simulink model "gm_dac_spi"  (R2022a)
settings: Solver=FixedStepDiscrete  StartTime=0.0  StopTime=1000/100e6  RelTol=1e-3
libraries: hdlsllib x152, simulink x1
settings Model: Creator=ts  LastModifiedBy=ts
settings SolverCC: AlgebraicLoopSolver=TrustRegion
settings DataIOCC: LimitDataPoints=on  SaveOutput=off  SaveTime=off
settings OptimizationCC: BlockReduction=off  ConditionallyExecuteInputs=off  DefaultParameterBehavior=Inlined  LifeSpan=inf
settings DebuggingCC: AlgebraicLoopMsg=error  InheritedTsInSrcMsg=none  SingleTaskRateTransMsg=error  UnconnectedInputMsg=warning  UnconnectedOutputMsg=warning  UnconnectedLineMsg=warning  AllowSymbolicDim=off  StrictBusMsg=ErrorOnBusTreatedAsVector  SFUnexpectedBacktrackingDiag=warning  SFNoUnconditionalDefaultTransitionDiag=warning  SFExecutionAtInitializationDiag=none  SFMachineParentedDataDiag=warning  ArithmeticOperatorsInVariantConditions=warning
settings HardwareCC: ProdBitPerPointer=32  ProdBitPerSizeT=32  ProdBitPerPtrDiffT=32  ProdLargestAtomicFloat=None  ProdIntDivRoundTo=Undefined  ProdEndianess=Unspecified  ProdWordSize=32  ProdHWDeviceType=ASIC/FPGA->ASIC/FPGA  ProdEqTarget=off
settings SFSimCC: SimUseLocalCustomCode=off  CustomCodeUndefinedFunction=UseInterfaceOnly
settings RTWCC: RTWUseLocalCustomCode=off
settings CodeAppCC: StateflowObjectComments=on
settings GRTTargetCC: TargetLangStandard=C89/C90 (ANSI)
settings ConfigComp: CovScope=ReferencedModels  CovMetricSettings=dw  CovSaveCumulativeToWorkspaceVar=on  CovSaveSingleToWorkspaceVar=on  CovExternalEMLEnable=off  CovSFcnEnable=off

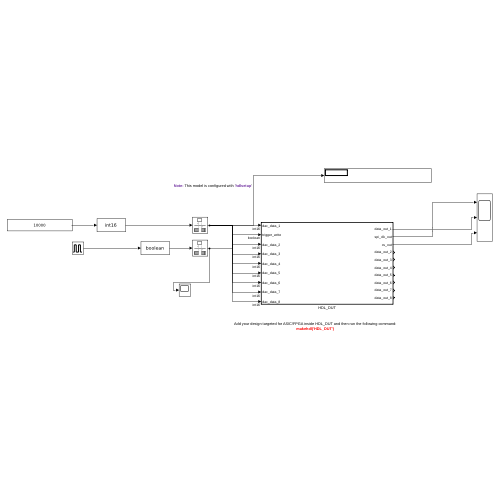
[thumbnail: Simulink's stored preview of the top-level diagram]
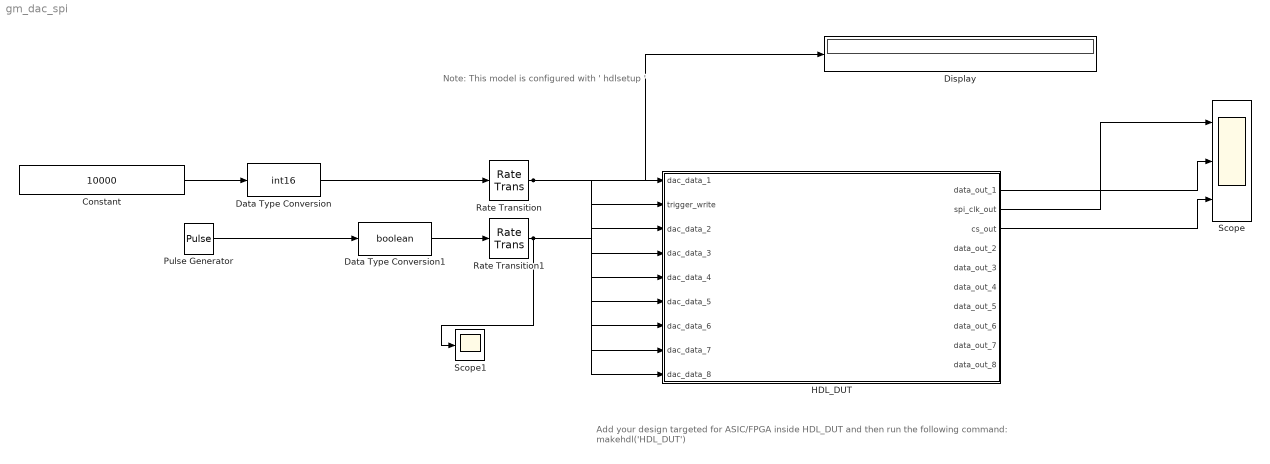
== system gm_dac_spi ==
  note: Add your design targeted for ASIC/FPGA inside HDL_DUT and then run the following command:
      | makehdl('HDL_DUT')
  note: Note: This model is configured with ' hdlsetup '
  Constant : Constant  Value=10000  OutDataTypeStr=int16  SampleTime=1/100e6
  Data Type Conversion : DataTypeConversion  OutDataTypeStr=int16  SaturateOnIntegerOverflow=off  RndMeth=Floor
  Data Type Conversion1 : DataTypeConversion  OutDataTypeStr=boolean  SaturateOnIntegerOverflow=off  RndMeth=Floor
  Display : Display
      settings: Format=binary (Stored Integer)
  HDL_DUT : Subsystem  TreatAsAtomicUnit=on
  Pulse Generator : DiscretePulseGenerator  PulseType=Time based  Period=200/100e6  PulseWidth=10
  Rate Transition : RateTransition  OutPortSampleTime=1/100e6
  Rate Transition1 : RateTransition  OutPortSampleTime=1/100e6
  Scope : Scope  NumInputPorts=3
  Scope1 : Scope
  wires:
  Pulse Generator/1 -> Data Type Conversion1/1
  Data Type Conversion1/1 -> Rate Transition1/1
  Rate Transition1/1 -> HDL_DUT/2(trigger_write), Scope1/1
  HDL_DUT/2(spi_clk_out) -> Scope/1
  HDL_DUT/3(cs_out) -> Scope/3
  Rate Transition/1 -> HDL_DUT/1(dac_data_1), HDL_DUT/3(dac_data_2), HDL_DUT/4(dac_data_3), HDL_DUT/5(dac_data_4), HDL_DUT/6(dac_data_5), HDL_DUT/7(dac_data_6), HDL_DUT/8(dac_data_7), HDL_DUT/9(dac_data_8), Display/1
  Data Type Conversion/1 -> Rate Transition/1
  HDL_DUT/1(data_out_1) -> Scope/2
  Constant/1 -> Data Type Conversion/1

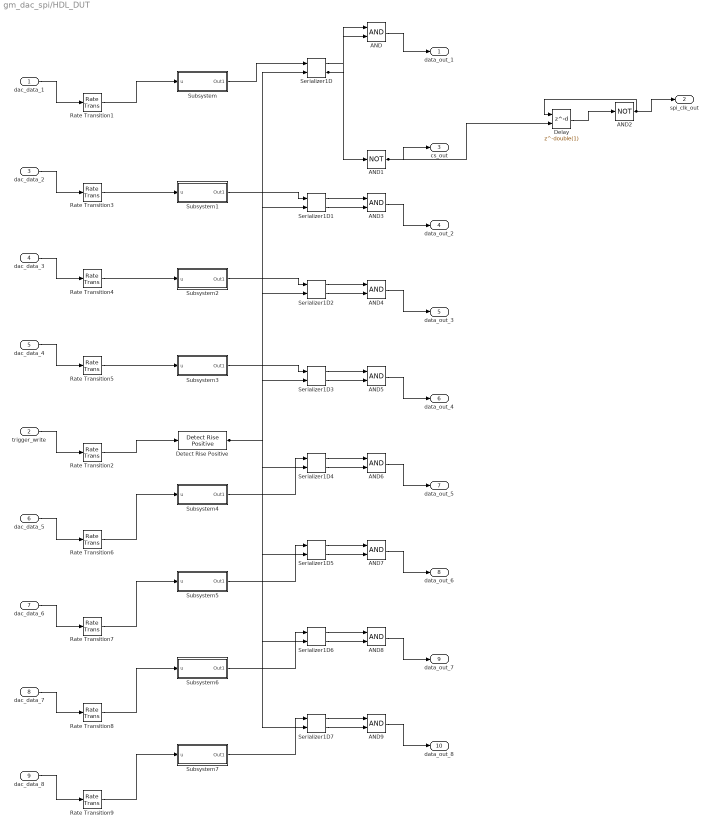
== system gm_dac_spi/HDL_DUT ==
  dac_data_1 : Inport  OutDataTypeStr=int16  PortDimensions=1  SampleTime=1e-08
  trigger_write : Inport  Port=2  OutDataTypeStr=boolean  PortDimensions=1  SampleTime=1e-08
  dac_data_2 : Inport  Port=3  OutDataTypeStr=int16  PortDimensions=1  SampleTime=1e-08
  dac_data_3 : Inport  Port=4  OutDataTypeStr=int16  PortDimensions=1  SampleTime=1e-08
  dac_data_4 : Inport  Port=5  OutDataTypeStr=int16  PortDimensions=1  SampleTime=1e-08
  dac_data_5 : Inport  Port=6  OutDataTypeStr=int16  PortDimensions=1  SampleTime=1e-08
  dac_data_6 : Inport  Port=7  OutDataTypeStr=int16  PortDimensions=1  SampleTime=1e-08
  dac_data_7 : Inport  Port=8  OutDataTypeStr=int16  PortDimensions=1  SampleTime=1e-08
  dac_data_8 : Inport  Port=9  OutDataTypeStr=int16  PortDimensions=1  SampleTime=1e-08
  AND{,3..9} (8 alike) : Logic  AllPortsSameDT=off  OutDataTypeStr=boolean  SampleTime=1e-08
  AND1 : Logic  Operator=NOT  Inputs=1  AllPortsSameDT=off  OutDataTypeStr=boolean  SampleTime=1e-08
  AND2 : Logic  Operator=NOT  Inputs=1  AllPortsSameDT=off  OutDataTypeStr=boolean  SampleTime=1e-08
  Delay : Delay  DelayLength=double(1)  InitialCondition=1  ExternalReset=Level
      settings: InputPortMap=u0,r5
  Detect Rise Positive : simulink/Logic and Bit Operations/Detect Rise Positive  vinit=0  OutDataTypeStr=boolean
  Rate Transition{1..9} (9 alike) : RateTransition  InitialCondition=double(0)  OutPortSampleTimeOpt=Multiple of input port sample time  OutPortSampleTimeMultiple=32
  Serializer1D{,1..7} (8 alike) : hdlsllib/HDL Operations/Serializer1D  Ratio=32  IdleCycles=0  validIn=on  startOut=off  validOut=on  inputDataDimensions=32  inputSampleTime=3.2e-07  inputSignalType=real
      settings: SourceProductBaseCode=SL
  Subsystem : Subsystem
  Subsystem1 : Subsystem
  Subsystem2 : Subsystem
  Subsystem3 : Subsystem
  Subsystem4 : Subsystem
  Subsystem5 : Subsystem
  Subsystem6 : Subsystem
  Subsystem7 : Subsystem
  data_out_1 : Outport  SampleTime=1e-08  VectorParamsAs1DForOutWhenUnconnected=off
  spi_clk_out : Outport  Port=2  SampleTime=1e-08
  cs_out : Outport  Port=3  SampleTime=1e-08
  data_out_2 : Outport  Port=4  SampleTime=1e-08  VectorParamsAs1DForOutWhenUnconnected=off
  data_out_3 : Outport  Port=5  SampleTime=1e-08  VectorParamsAs1DForOutWhenUnconnected=off
  data_out_4 : Outport  Port=6  SampleTime=1e-08  VectorParamsAs1DForOutWhenUnconnected=off
  data_out_5 : Outport  Port=7  SampleTime=1e-08  VectorParamsAs1DForOutWhenUnconnected=off
  data_out_6 : Outport  Port=8  SampleTime=1e-08  VectorParamsAs1DForOutWhenUnconnected=off
  data_out_7 : Outport  Port=9  SampleTime=1e-08  VectorParamsAs1DForOutWhenUnconnected=off
  data_out_8 : Outport  Port=10  SampleTime=1e-08  VectorParamsAs1DForOutWhenUnconnected=off
  wires:
  dac_data_1/1 -> Rate Transition1/1
  trigger_write/1 -> Rate Transition2/1
  dac_data_2/1 -> Rate Transition3/1
  dac_data_3/1 -> Rate Transition4/1
  dac_data_4/1 -> Rate Transition5/1
  dac_data_5/1 -> Rate Transition6/1
  dac_data_6/1 -> Rate Transition7/1
  dac_data_7/1 -> Rate Transition8/1
  dac_data_8/1 -> Rate Transition9/1
  AND/1 -> data_out_1/1
  AND1/1 -> Delay/2, cs_out/1
  AND2/1 -> Delay/1, spi_clk_out/1
  AND3/1 -> data_out_2/1
  AND4/1 -> data_out_3/1
  AND5/1 -> data_out_4/1
  AND6/1 -> data_out_5/1
  AND7/1 -> data_out_6/1
  AND8/1 -> data_out_7/1
  AND9/1 -> data_out_8/1
  Delay/1 -> AND2/1
  Detect Rise Positive/1 -> Serializer1D7/2, Serializer1D6/2, Serializer1D5/2, Serializer1D4/2, Serializer1D3/2, Serializer1D2/2, Serializer1D1/2, Serializer1D/2
  Rate Transition1/1 -> Subsystem/1(u)
  Rate Transition2/1 -> Detect Rise Positive/1
  Rate Transition3/1 -> Subsystem1/1(u)
  Rate Transition4/1 -> Subsystem2/1(u)
  Rate Transition5/1 -> Subsystem3/1(u)
  Rate Transition6/1 -> Subsystem4/1(u)
  Rate Transition7/1 -> Subsystem5/1(u)
  Rate Transition8/1 -> Subsystem6/1(u)
  Rate Transition9/1 -> Subsystem7/1(u)
  Serializer1D/1 -> AND/1
  Serializer1D/2 -> AND1/1, AND/2
  Serializer1D1/1 -> AND3/1
  Serializer1D1/2 -> AND3/2
  Serializer1D2/1 -> AND4/1
  Serializer1D2/2 -> AND4/2
  Serializer1D3/1 -> AND5/1
  Serializer1D3/2 -> AND5/2
  Serializer1D4/1 -> AND6/1
  Serializer1D4/2 -> AND6/2
  Serializer1D5/1 -> AND7/1
  Serializer1D5/2 -> AND7/2
  Serializer1D6/1 -> AND8/1
  Serializer1D6/2 -> AND8/2
  Serializer1D7/1 -> AND9/1
  Serializer1D7/2 -> AND9/2
  Subsystem/1(Out1) -> Serializer1D/1
  Subsystem1/1(Out1) -> Serializer1D1/1
  Subsystem2/1(Out1) -> Serializer1D2/1
  Subsystem3/1(Out1) -> Serializer1D3/1
  Subsystem4/1(Out1) -> Serializer1D4/1
  Subsystem5/1(Out1) -> Serializer1D5/1
  Subsystem6/1(Out1) -> Serializer1D6/1
  Subsystem7/1(Out1) -> Serializer1D7/1

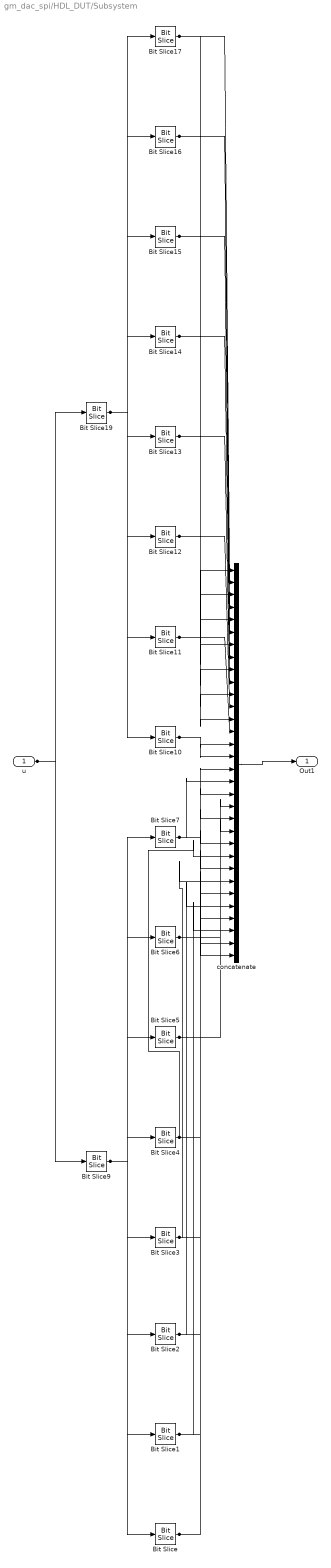
== system gm_dac_spi/HDL_DUT/Subsystem ==
  u : Inport  OutDataTypeStr=int16  PortDimensions=1  SampleTime=3.2e-07
  Bit Slice : hdlsllib/Logic and Bit Operations/Bit Slice  lidx=double(0)  ridx=double(0)
      settings: SourceProductBaseCode=SL
  Bit Slice1 : hdlsllib/Logic and Bit Operations/Bit Slice  lidx=double(1)  ridx=double(1)
      settings: SourceProductBaseCode=SL
  Bit Slice10 : hdlsllib/Logic and Bit Operations/Bit Slice  lidx=double(0)  ridx=double(0)
      settings: SourceProductBaseCode=SL
  Bit Slice11 : hdlsllib/Logic and Bit Operations/Bit Slice  lidx=double(1)  ridx=double(1)
      settings: SourceProductBaseCode=SL
  Bit Slice12 : hdlsllib/Logic and Bit Operations/Bit Slice  lidx=double(2)  ridx=double(2)
      settings: SourceProductBaseCode=SL
  Bit Slice13 : hdlsllib/Logic and Bit Operations/Bit Slice  lidx=double(3)  ridx=double(3)
      settings: SourceProductBaseCode=SL
  Bit Slice14 : hdlsllib/Logic and Bit Operations/Bit Slice  lidx=double(4)  ridx=double(4)
      settings: SourceProductBaseCode=SL
  Bit Slice15 : hdlsllib/Logic and Bit Operations/Bit Slice  lidx=double(5)  ridx=double(5)
      settings: SourceProductBaseCode=SL
  Bit Slice16 : hdlsllib/Logic and Bit Operations/Bit Slice  lidx=double(6)  ridx=double(6)
      settings: SourceProductBaseCode=SL
  Bit Slice17 : hdlsllib/Logic and Bit Operations/Bit Slice  lidx=double(7)  ridx=double(7)
      settings: SourceProductBaseCode=SL
  Bit Slice19 : hdlsllib/Logic and Bit Operations/Bit Slice  lidx=double(15)  ridx=double(8)
      settings: SourceProductBaseCode=SL
  Bit Slice2 : hdlsllib/Logic and Bit Operations/Bit Slice  lidx=double(2)  ridx=double(2)
      settings: SourceProductBaseCode=SL
  Bit Slice3 : hdlsllib/Logic and Bit Operations/Bit Slice  lidx=double(3)  ridx=double(3)
      settings: SourceProductBaseCode=SL
  Bit Slice4 : hdlsllib/Logic and Bit Operations/Bit Slice  lidx=double(4)  ridx=double(4)
      settings: SourceProductBaseCode=SL
  Bit Slice5 : hdlsllib/Logic and Bit Operations/Bit Slice  lidx=double(5)  ridx=double(5)
      settings: SourceProductBaseCode=SL
  Bit Slice6 : hdlsllib/Logic and Bit Operations/Bit Slice  lidx=double(6)  ridx=double(6)
      settings: SourceProductBaseCode=SL
  Bit Slice7 : hdlsllib/Logic and Bit Operations/Bit Slice  lidx=double(7)  ridx=double(7)
      settings: SourceProductBaseCode=SL
  Bit Slice9 : hdlsllib/Logic and Bit Operations/Bit Slice  lidx=double(7)  ridx=double(0)
      settings: SourceProductBaseCode=SL
  concatenate : Concatenate  NumInputs=32
  Out1 : Outport  SampleTime=3.2e-07
  wires:
  u/1 -> Bit Slice9/1, Bit Slice19/1
  Bit Slice/1 -> concatenate/32, concatenate/31
  Bit Slice1/1 -> concatenate/30, concatenate/29
  Bit Slice10/1 -> concatenate/16, concatenate/15
  Bit Slice11/1 -> concatenate/14, concatenate/13
  Bit Slice12/1 -> concatenate/12, concatenate/11
  Bit Slice13/1 -> concatenate/10, concatenate/9
  Bit Slice14/1 -> concatenate/8, concatenate/7
  Bit Slice15/1 -> concatenate/6, concatenate/5
  Bit Slice16/1 -> concatenate/4, concatenate/3
  Bit Slice17/1 -> concatenate/2, concatenate/1
  Bit Slice19/1 -> Bit Slice17/1, Bit Slice16/1, Bit Slice15/1, Bit Slice14/1, Bit Slice13/1, Bit Slice12/1, Bit Slice11/1, Bit Slice10/1
  Bit Slice2/1 -> concatenate/28, concatenate/27
  Bit Slice3/1 -> concatenate/26, concatenate/25
  Bit Slice4/1 -> concatenate/24, concatenate/23
  Bit Slice5/1 -> concatenate/22, concatenate/21
  Bit Slice6/1 -> concatenate/20, concatenate/19
  Bit Slice7/1 -> concatenate/18, concatenate/17
  Bit Slice9/1 -> Bit Slice7/1, Bit Slice6/1, Bit Slice5/1, Bit Slice4/1, Bit Slice3/1, Bit Slice2/1, Bit Slice1/1, Bit Slice/1
  concatenate/1 -> Out1/1

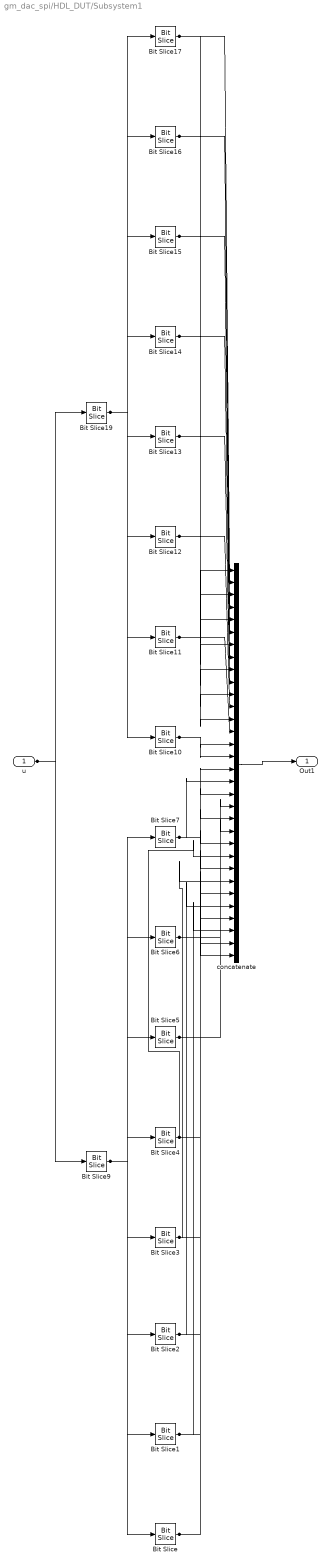
== system gm_dac_spi/HDL_DUT/Subsystem1 ==
  u : Inport  OutDataTypeStr=int16  PortDimensions=1  SampleTime=3.2e-07
  Bit Slice : hdlsllib/Logic and Bit Operations/Bit Slice  lidx=double(0)  ridx=double(0)
      settings: SourceProductBaseCode=SL
  Bit Slice1 : hdlsllib/Logic and Bit Operations/Bit Slice  lidx=double(1)  ridx=double(1)
      settings: SourceProductBaseCode=SL
  Bit Slice10 : hdlsllib/Logic and Bit Operations/Bit Slice  lidx=double(0)  ridx=double(0)
      settings: SourceProductBaseCode=SL
  Bit Slice11 : hdlsllib/Logic and Bit Operations/Bit Slice  lidx=double(1)  ridx=double(1)
      settings: SourceProductBaseCode=SL
  Bit Slice12 : hdlsllib/Logic and Bit Operations/Bit Slice  lidx=double(2)  ridx=double(2)
      settings: SourceProductBaseCode=SL
  Bit Slice13 : hdlsllib/Logic and Bit Operations/Bit Slice  lidx=double(3)  ridx=double(3)
      settings: SourceProductBaseCode=SL
  Bit Slice14 : hdlsllib/Logic and Bit Operations/Bit Slice  lidx=double(4)  ridx=double(4)
      settings: SourceProductBaseCode=SL
  Bit Slice15 : hdlsllib/Logic and Bit Operations/Bit Slice  lidx=double(5)  ridx=double(5)
      settings: SourceProductBaseCode=SL
  Bit Slice16 : hdlsllib/Logic and Bit Operations/Bit Slice  lidx=double(6)  ridx=double(6)
      settings: SourceProductBaseCode=SL
  Bit Slice17 : hdlsllib/Logic and Bit Operations/Bit Slice  lidx=double(7)  ridx=double(7)
      settings: SourceProductBaseCode=SL
  Bit Slice19 : hdlsllib/Logic and Bit Operations/Bit Slice  lidx=double(15)  ridx=double(8)
      settings: SourceProductBaseCode=SL
  Bit Slice2 : hdlsllib/Logic and Bit Operations/Bit Slice  lidx=double(2)  ridx=double(2)
      settings: SourceProductBaseCode=SL
  Bit Slice3 : hdlsllib/Logic and Bit Operations/Bit Slice  lidx=double(3)  ridx=double(3)
      settings: SourceProductBaseCode=SL
  Bit Slice4 : hdlsllib/Logic and Bit Operations/Bit Slice  lidx=double(4)  ridx=double(4)
      settings: SourceProductBaseCode=SL
  Bit Slice5 : hdlsllib/Logic and Bit Operations/Bit Slice  lidx=double(5)  ridx=double(5)
      settings: SourceProductBaseCode=SL
  Bit Slice6 : hdlsllib/Logic and Bit Operations/Bit Slice  lidx=double(6)  ridx=double(6)
      settings: SourceProductBaseCode=SL
  Bit Slice7 : hdlsllib/Logic and Bit Operations/Bit Slice  lidx=double(7)  ridx=double(7)
      settings: SourceProductBaseCode=SL
  Bit Slice9 : hdlsllib/Logic and Bit Operations/Bit Slice  lidx=double(7)  ridx=double(0)
      settings: SourceProductBaseCode=SL
  concatenate : Concatenate  NumInputs=32
  Out1 : Outport  SampleTime=3.2e-07
  wires:
  u/1 -> Bit Slice9/1, Bit Slice19/1
  Bit Slice/1 -> concatenate/32, concatenate/31
  Bit Slice1/1 -> concatenate/30, concatenate/29
  Bit Slice10/1 -> concatenate/16, concatenate/15
  Bit Slice11/1 -> concatenate/14, concatenate/13
  Bit Slice12/1 -> concatenate/12, concatenate/11
  Bit Slice13/1 -> concatenate/10, concatenate/9
  Bit Slice14/1 -> concatenate/8, concatenate/7
  Bit Slice15/1 -> concatenate/6, concatenate/5
  Bit Slice16/1 -> concatenate/4, concatenate/3
  Bit Slice17/1 -> concatenate/2, concatenate/1
  Bit Slice19/1 -> Bit Slice17/1, Bit Slice16/1, Bit Slice15/1, Bit Slice14/1, Bit Slice13/1, Bit Slice12/1, Bit Slice11/1, Bit Slice10/1
  Bit Slice2/1 -> concatenate/28, concatenate/27
  Bit Slice3/1 -> concatenate/26, concatenate/25
  Bit Slice4/1 -> concatenate/24, concatenate/23
  Bit Slice5/1 -> concatenate/22, concatenate/21
  Bit Slice6/1 -> concatenate/20, concatenate/19
  Bit Slice7/1 -> concatenate/18, concatenate/17
  Bit Slice9/1 -> Bit Slice7/1, Bit Slice6/1, Bit Slice5/1, Bit Slice4/1, Bit Slice3/1, Bit Slice2/1, Bit Slice1/1, Bit Slice/1
  concatenate/1 -> Out1/1

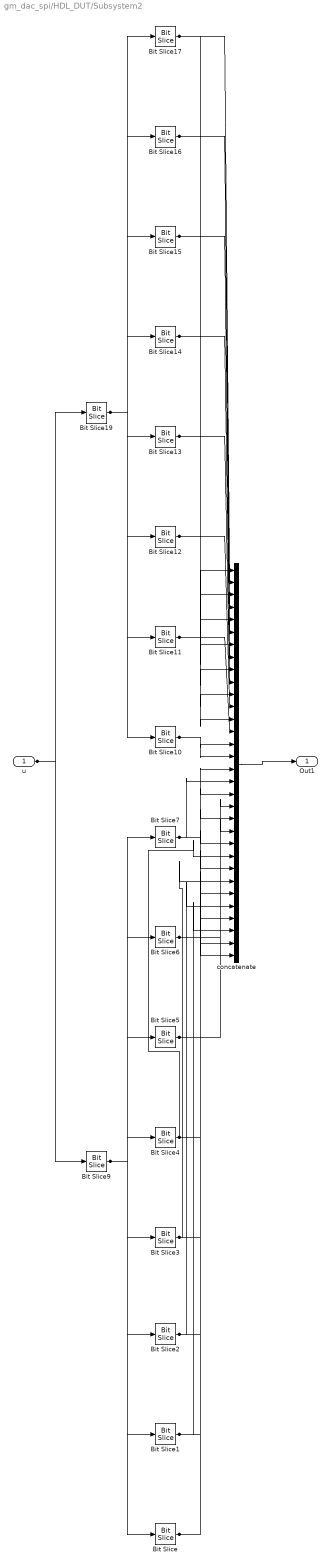
== system gm_dac_spi/HDL_DUT/Subsystem2 ==
  u : Inport  OutDataTypeStr=int16  PortDimensions=1  SampleTime=3.2e-07
  Bit Slice : hdlsllib/Logic and Bit Operations/Bit Slice  lidx=double(0)  ridx=double(0)
      settings: SourceProductBaseCode=SL
  Bit Slice1 : hdlsllib/Logic and Bit Operations/Bit Slice  lidx=double(1)  ridx=double(1)
      settings: SourceProductBaseCode=SL
  Bit Slice10 : hdlsllib/Logic and Bit Operations/Bit Slice  lidx=double(0)  ridx=double(0)
      settings: SourceProductBaseCode=SL
  Bit Slice11 : hdlsllib/Logic and Bit Operations/Bit Slice  lidx=double(1)  ridx=double(1)
      settings: SourceProductBaseCode=SL
  Bit Slice12 : hdlsllib/Logic and Bit Operations/Bit Slice  lidx=double(2)  ridx=double(2)
      settings: SourceProductBaseCode=SL
  Bit Slice13 : hdlsllib/Logic and Bit Operations/Bit Slice  lidx=double(3)  ridx=double(3)
      settings: SourceProductBaseCode=SL
  Bit Slice14 : hdlsllib/Logic and Bit Operations/Bit Slice  lidx=double(4)  ridx=double(4)
      settings: SourceProductBaseCode=SL
  Bit Slice15 : hdlsllib/Logic and Bit Operations/Bit Slice  lidx=double(5)  ridx=double(5)
      settings: SourceProductBaseCode=SL
  Bit Slice16 : hdlsllib/Logic and Bit Operations/Bit Slice  lidx=double(6)  ridx=double(6)
      settings: SourceProductBaseCode=SL
  Bit Slice17 : hdlsllib/Logic and Bit Operations/Bit Slice  lidx=double(7)  ridx=double(7)
      settings: SourceProductBaseCode=SL
  Bit Slice19 : hdlsllib/Logic and Bit Operations/Bit Slice  lidx=double(15)  ridx=double(8)
      settings: SourceProductBaseCode=SL
  Bit Slice2 : hdlsllib/Logic and Bit Operations/Bit Slice  lidx=double(2)  ridx=double(2)
      settings: SourceProductBaseCode=SL
  Bit Slice3 : hdlsllib/Logic and Bit Operations/Bit Slice  lidx=double(3)  ridx=double(3)
      settings: SourceProductBaseCode=SL
  Bit Slice4 : hdlsllib/Logic and Bit Operations/Bit Slice  lidx=double(4)  ridx=double(4)
      settings: SourceProductBaseCode=SL
  Bit Slice5 : hdlsllib/Logic and Bit Operations/Bit Slice  lidx=double(5)  ridx=double(5)
      settings: SourceProductBaseCode=SL
  Bit Slice6 : hdlsllib/Logic and Bit Operations/Bit Slice  lidx=double(6)  ridx=double(6)
      settings: SourceProductBaseCode=SL
  Bit Slice7 : hdlsllib/Logic and Bit Operations/Bit Slice  lidx=double(7)  ridx=double(7)
      settings: SourceProductBaseCode=SL
  Bit Slice9 : hdlsllib/Logic and Bit Operations/Bit Slice  lidx=double(7)  ridx=double(0)
      settings: SourceProductBaseCode=SL
  concatenate : Concatenate  NumInputs=32
  Out1 : Outport  SampleTime=3.2e-07
  wires:
  u/1 -> Bit Slice9/1, Bit Slice19/1
  Bit Slice/1 -> concatenate/32, concatenate/31
  Bit Slice1/1 -> concatenate/30, concatenate/29
  Bit Slice10/1 -> concatenate/16, concatenate/15
  Bit Slice11/1 -> concatenate/14, concatenate/13
  Bit Slice12/1 -> concatenate/12, concatenate/11
  Bit Slice13/1 -> concatenate/10, concatenate/9
  Bit Slice14/1 -> concatenate/8, concatenate/7
  Bit Slice15/1 -> concatenate/6, concatenate/5
  Bit Slice16/1 -> concatenate/4, concatenate/3
  Bit Slice17/1 -> concatenate/2, concatenate/1
  Bit Slice19/1 -> Bit Slice17/1, Bit Slice16/1, Bit Slice15/1, Bit Slice14/1, Bit Slice13/1, Bit Slice12/1, Bit Slice11/1, Bit Slice10/1
  Bit Slice2/1 -> concatenate/28, concatenate/27
  Bit Slice3/1 -> concatenate/26, concatenate/25
  Bit Slice4/1 -> concatenate/24, concatenate/23
  Bit Slice5/1 -> concatenate/22, concatenate/21
  Bit Slice6/1 -> concatenate/20, concatenate/19
  Bit Slice7/1 -> concatenate/18, concatenate/17
  Bit Slice9/1 -> Bit Slice7/1, Bit Slice6/1, Bit Slice5/1, Bit Slice4/1, Bit Slice3/1, Bit Slice2/1, Bit Slice1/1, Bit Slice/1
  concatenate/1 -> Out1/1

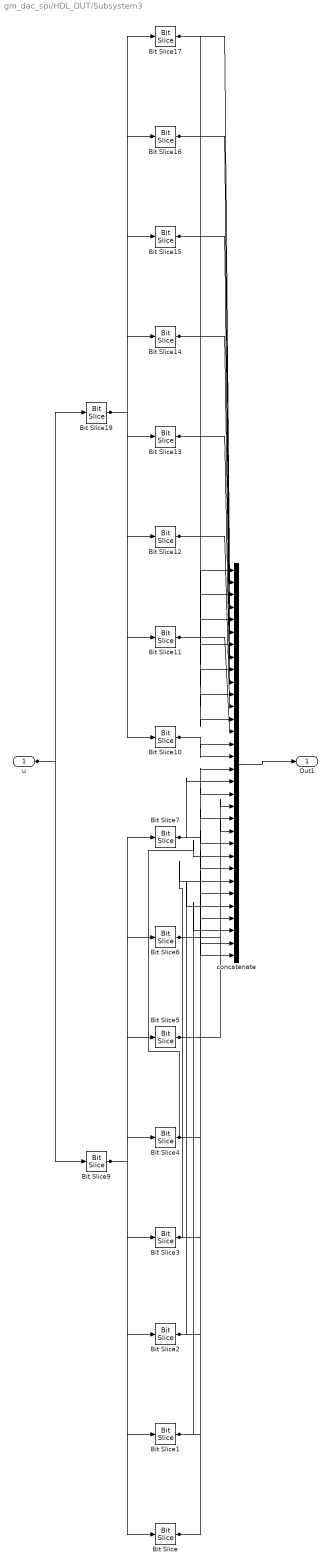
== system gm_dac_spi/HDL_DUT/Subsystem3 ==
  u : Inport  OutDataTypeStr=int16  PortDimensions=1  SampleTime=3.2e-07
  Bit Slice : hdlsllib/Logic and Bit Operations/Bit Slice  lidx=double(0)  ridx=double(0)
      settings: SourceProductBaseCode=SL
  Bit Slice1 : hdlsllib/Logic and Bit Operations/Bit Slice  lidx=double(1)  ridx=double(1)
      settings: SourceProductBaseCode=SL
  Bit Slice10 : hdlsllib/Logic and Bit Operations/Bit Slice  lidx=double(0)  ridx=double(0)
      settings: SourceProductBaseCode=SL
  Bit Slice11 : hdlsllib/Logic and Bit Operations/Bit Slice  lidx=double(1)  ridx=double(1)
      settings: SourceProductBaseCode=SL
  Bit Slice12 : hdlsllib/Logic and Bit Operations/Bit Slice  lidx=double(2)  ridx=double(2)
      settings: SourceProductBaseCode=SL
  Bit Slice13 : hdlsllib/Logic and Bit Operations/Bit Slice  lidx=double(3)  ridx=double(3)
      settings: SourceProductBaseCode=SL
  Bit Slice14 : hdlsllib/Logic and Bit Operations/Bit Slice  lidx=double(4)  ridx=double(4)
      settings: SourceProductBaseCode=SL
  Bit Slice15 : hdlsllib/Logic and Bit Operations/Bit Slice  lidx=double(5)  ridx=double(5)
      settings: SourceProductBaseCode=SL
  Bit Slice16 : hdlsllib/Logic and Bit Operations/Bit Slice  lidx=double(6)  ridx=double(6)
      settings: SourceProductBaseCode=SL
  Bit Slice17 : hdlsllib/Logic and Bit Operations/Bit Slice  lidx=double(7)  ridx=double(7)
      settings: SourceProductBaseCode=SL
  Bit Slice19 : hdlsllib/Logic and Bit Operations/Bit Slice  lidx=double(15)  ridx=double(8)
      settings: SourceProductBaseCode=SL
  Bit Slice2 : hdlsllib/Logic and Bit Operations/Bit Slice  lidx=double(2)  ridx=double(2)
      settings: SourceProductBaseCode=SL
  Bit Slice3 : hdlsllib/Logic and Bit Operations/Bit Slice  lidx=double(3)  ridx=double(3)
      settings: SourceProductBaseCode=SL
  Bit Slice4 : hdlsllib/Logic and Bit Operations/Bit Slice  lidx=double(4)  ridx=double(4)
      settings: SourceProductBaseCode=SL
  Bit Slice5 : hdlsllib/Logic and Bit Operations/Bit Slice  lidx=double(5)  ridx=double(5)
      settings: SourceProductBaseCode=SL
  Bit Slice6 : hdlsllib/Logic and Bit Operations/Bit Slice  lidx=double(6)  ridx=double(6)
      settings: SourceProductBaseCode=SL
  Bit Slice7 : hdlsllib/Logic and Bit Operations/Bit Slice  lidx=double(7)  ridx=double(7)
      settings: SourceProductBaseCode=SL
  Bit Slice9 : hdlsllib/Logic and Bit Operations/Bit Slice  lidx=double(7)  ridx=double(0)
      settings: SourceProductBaseCode=SL
  concatenate : Concatenate  NumInputs=32
  Out1 : Outport  SampleTime=3.2e-07
  wires:
  u/1 -> Bit Slice9/1, Bit Slice19/1
  Bit Slice/1 -> concatenate/32, concatenate/31
  Bit Slice1/1 -> concatenate/30, concatenate/29
  Bit Slice10/1 -> concatenate/16, concatenate/15
  Bit Slice11/1 -> concatenate/14, concatenate/13
  Bit Slice12/1 -> concatenate/12, concatenate/11
  Bit Slice13/1 -> concatenate/10, concatenate/9
  Bit Slice14/1 -> concatenate/8, concatenate/7
  Bit Slice15/1 -> concatenate/6, concatenate/5
  Bit Slice16/1 -> concatenate/4, concatenate/3
  Bit Slice17/1 -> concatenate/2, concatenate/1
  Bit Slice19/1 -> Bit Slice17/1, Bit Slice16/1, Bit Slice15/1, Bit Slice14/1, Bit Slice13/1, Bit Slice12/1, Bit Slice11/1, Bit Slice10/1
  Bit Slice2/1 -> concatenate/28, concatenate/27
  Bit Slice3/1 -> concatenate/26, concatenate/25
  Bit Slice4/1 -> concatenate/24, concatenate/23
  Bit Slice5/1 -> concatenate/22, concatenate/21
  Bit Slice6/1 -> concatenate/20, concatenate/19
  Bit Slice7/1 -> concatenate/18, concatenate/17
  Bit Slice9/1 -> Bit Slice7/1, Bit Slice6/1, Bit Slice5/1, Bit Slice4/1, Bit Slice3/1, Bit Slice2/1, Bit Slice1/1, Bit Slice/1
  concatenate/1 -> Out1/1

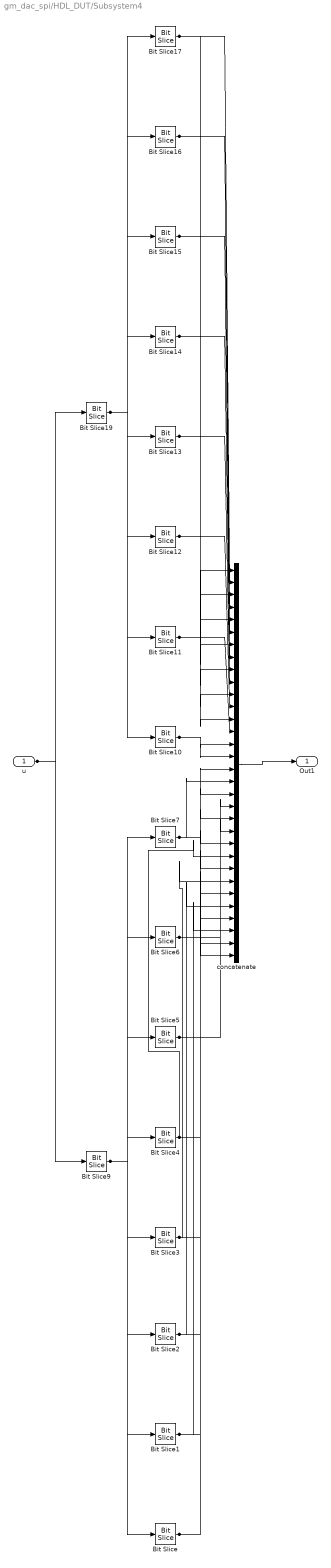
== system gm_dac_spi/HDL_DUT/Subsystem4 ==
  u : Inport  OutDataTypeStr=int16  PortDimensions=1  SampleTime=3.2e-07
  Bit Slice : hdlsllib/Logic and Bit Operations/Bit Slice  lidx=double(0)  ridx=double(0)
      settings: SourceProductBaseCode=SL
  Bit Slice1 : hdlsllib/Logic and Bit Operations/Bit Slice  lidx=double(1)  ridx=double(1)
      settings: SourceProductBaseCode=SL
  Bit Slice10 : hdlsllib/Logic and Bit Operations/Bit Slice  lidx=double(0)  ridx=double(0)
      settings: SourceProductBaseCode=SL
  Bit Slice11 : hdlsllib/Logic and Bit Operations/Bit Slice  lidx=double(1)  ridx=double(1)
      settings: SourceProductBaseCode=SL
  Bit Slice12 : hdlsllib/Logic and Bit Operations/Bit Slice  lidx=double(2)  ridx=double(2)
      settings: SourceProductBaseCode=SL
  Bit Slice13 : hdlsllib/Logic and Bit Operations/Bit Slice  lidx=double(3)  ridx=double(3)
      settings: SourceProductBaseCode=SL
  Bit Slice14 : hdlsllib/Logic and Bit Operations/Bit Slice  lidx=double(4)  ridx=double(4)
      settings: SourceProductBaseCode=SL
  Bit Slice15 : hdlsllib/Logic and Bit Operations/Bit Slice  lidx=double(5)  ridx=double(5)
      settings: SourceProductBaseCode=SL
  Bit Slice16 : hdlsllib/Logic and Bit Operations/Bit Slice  lidx=double(6)  ridx=double(6)
      settings: SourceProductBaseCode=SL
  Bit Slice17 : hdlsllib/Logic and Bit Operations/Bit Slice  lidx=double(7)  ridx=double(7)
      settings: SourceProductBaseCode=SL
  Bit Slice19 : hdlsllib/Logic and Bit Operations/Bit Slice  lidx=double(15)  ridx=double(8)
      settings: SourceProductBaseCode=SL
  Bit Slice2 : hdlsllib/Logic and Bit Operations/Bit Slice  lidx=double(2)  ridx=double(2)
      settings: SourceProductBaseCode=SL
  Bit Slice3 : hdlsllib/Logic and Bit Operations/Bit Slice  lidx=double(3)  ridx=double(3)
      settings: SourceProductBaseCode=SL
  Bit Slice4 : hdlsllib/Logic and Bit Operations/Bit Slice  lidx=double(4)  ridx=double(4)
      settings: SourceProductBaseCode=SL
  Bit Slice5 : hdlsllib/Logic and Bit Operations/Bit Slice  lidx=double(5)  ridx=double(5)
      settings: SourceProductBaseCode=SL
  Bit Slice6 : hdlsllib/Logic and Bit Operations/Bit Slice  lidx=double(6)  ridx=double(6)
      settings: SourceProductBaseCode=SL
  Bit Slice7 : hdlsllib/Logic and Bit Operations/Bit Slice  lidx=double(7)  ridx=double(7)
      settings: SourceProductBaseCode=SL
  Bit Slice9 : hdlsllib/Logic and Bit Operations/Bit Slice  lidx=double(7)  ridx=double(0)
      settings: SourceProductBaseCode=SL
  concatenate : Concatenate  NumInputs=32
  Out1 : Outport  SampleTime=3.2e-07
  wires:
  u/1 -> Bit Slice9/1, Bit Slice19/1
  Bit Slice/1 -> concatenate/32, concatenate/31
  Bit Slice1/1 -> concatenate/30, concatenate/29
  Bit Slice10/1 -> concatenate/16, concatenate/15
  Bit Slice11/1 -> concatenate/14, concatenate/13
  Bit Slice12/1 -> concatenate/12, concatenate/11
  Bit Slice13/1 -> concatenate/10, concatenate/9
  Bit Slice14/1 -> concatenate/8, concatenate/7
  Bit Slice15/1 -> concatenate/6, concatenate/5
  Bit Slice16/1 -> concatenate/4, concatenate/3
  Bit Slice17/1 -> concatenate/2, concatenate/1
  Bit Slice19/1 -> Bit Slice17/1, Bit Slice16/1, Bit Slice15/1, Bit Slice14/1, Bit Slice13/1, Bit Slice12/1, Bit Slice11/1, Bit Slice10/1
  Bit Slice2/1 -> concatenate/28, concatenate/27
  Bit Slice3/1 -> concatenate/26, concatenate/25
  Bit Slice4/1 -> concatenate/24, concatenate/23
  Bit Slice5/1 -> concatenate/22, concatenate/21
  Bit Slice6/1 -> concatenate/20, concatenate/19
  Bit Slice7/1 -> concatenate/18, concatenate/17
  Bit Slice9/1 -> Bit Slice7/1, Bit Slice6/1, Bit Slice5/1, Bit Slice4/1, Bit Slice3/1, Bit Slice2/1, Bit Slice1/1, Bit Slice/1
  concatenate/1 -> Out1/1

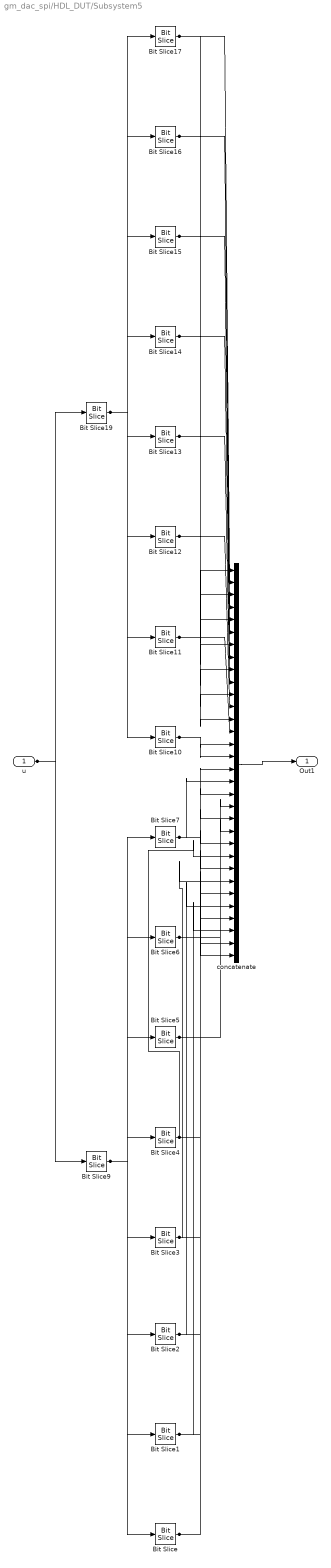
== system gm_dac_spi/HDL_DUT/Subsystem5 ==
  u : Inport  OutDataTypeStr=int16  PortDimensions=1  SampleTime=3.2e-07
  Bit Slice : hdlsllib/Logic and Bit Operations/Bit Slice  lidx=double(0)  ridx=double(0)
      settings: SourceProductBaseCode=SL
  Bit Slice1 : hdlsllib/Logic and Bit Operations/Bit Slice  lidx=double(1)  ridx=double(1)
      settings: SourceProductBaseCode=SL
  Bit Slice10 : hdlsllib/Logic and Bit Operations/Bit Slice  lidx=double(0)  ridx=double(0)
      settings: SourceProductBaseCode=SL
  Bit Slice11 : hdlsllib/Logic and Bit Operations/Bit Slice  lidx=double(1)  ridx=double(1)
      settings: SourceProductBaseCode=SL
  Bit Slice12 : hdlsllib/Logic and Bit Operations/Bit Slice  lidx=double(2)  ridx=double(2)
      settings: SourceProductBaseCode=SL
  Bit Slice13 : hdlsllib/Logic and Bit Operations/Bit Slice  lidx=double(3)  ridx=double(3)
      settings: SourceProductBaseCode=SL
  Bit Slice14 : hdlsllib/Logic and Bit Operations/Bit Slice  lidx=double(4)  ridx=double(4)
      settings: SourceProductBaseCode=SL
  Bit Slice15 : hdlsllib/Logic and Bit Operations/Bit Slice  lidx=double(5)  ridx=double(5)
      settings: SourceProductBaseCode=SL
  Bit Slice16 : hdlsllib/Logic and Bit Operations/Bit Slice  lidx=double(6)  ridx=double(6)
      settings: SourceProductBaseCode=SL
  Bit Slice17 : hdlsllib/Logic and Bit Operations/Bit Slice  lidx=double(7)  ridx=double(7)
      settings: SourceProductBaseCode=SL
  Bit Slice19 : hdlsllib/Logic and Bit Operations/Bit Slice  lidx=double(15)  ridx=double(8)
      settings: SourceProductBaseCode=SL
  Bit Slice2 : hdlsllib/Logic and Bit Operations/Bit Slice  lidx=double(2)  ridx=double(2)
      settings: SourceProductBaseCode=SL
  Bit Slice3 : hdlsllib/Logic and Bit Operations/Bit Slice  lidx=double(3)  ridx=double(3)
      settings: SourceProductBaseCode=SL
  Bit Slice4 : hdlsllib/Logic and Bit Operations/Bit Slice  lidx=double(4)  ridx=double(4)
      settings: SourceProductBaseCode=SL
  Bit Slice5 : hdlsllib/Logic and Bit Operations/Bit Slice  lidx=double(5)  ridx=double(5)
      settings: SourceProductBaseCode=SL
  Bit Slice6 : hdlsllib/Logic and Bit Operations/Bit Slice  lidx=double(6)  ridx=double(6)
      settings: SourceProductBaseCode=SL
  Bit Slice7 : hdlsllib/Logic and Bit Operations/Bit Slice  lidx=double(7)  ridx=double(7)
      settings: SourceProductBaseCode=SL
  Bit Slice9 : hdlsllib/Logic and Bit Operations/Bit Slice  lidx=double(7)  ridx=double(0)
      settings: SourceProductBaseCode=SL
  concatenate : Concatenate  NumInputs=32
  Out1 : Outport  SampleTime=3.2e-07
  wires:
  u/1 -> Bit Slice9/1, Bit Slice19/1
  Bit Slice/1 -> concatenate/32, concatenate/31
  Bit Slice1/1 -> concatenate/30, concatenate/29
  Bit Slice10/1 -> concatenate/16, concatenate/15
  Bit Slice11/1 -> concatenate/14, concatenate/13
  Bit Slice12/1 -> concatenate/12, concatenate/11
  Bit Slice13/1 -> concatenate/10, concatenate/9
  Bit Slice14/1 -> concatenate/8, concatenate/7
  Bit Slice15/1 -> concatenate/6, concatenate/5
  Bit Slice16/1 -> concatenate/4, concatenate/3
  Bit Slice17/1 -> concatenate/2, concatenate/1
  Bit Slice19/1 -> Bit Slice17/1, Bit Slice16/1, Bit Slice15/1, Bit Slice14/1, Bit Slice13/1, Bit Slice12/1, Bit Slice11/1, Bit Slice10/1
  Bit Slice2/1 -> concatenate/28, concatenate/27
  Bit Slice3/1 -> concatenate/26, concatenate/25
  Bit Slice4/1 -> concatenate/24, concatenate/23
  Bit Slice5/1 -> concatenate/22, concatenate/21
  Bit Slice6/1 -> concatenate/20, concatenate/19
  Bit Slice7/1 -> concatenate/18, concatenate/17
  Bit Slice9/1 -> Bit Slice7/1, Bit Slice6/1, Bit Slice5/1, Bit Slice4/1, Bit Slice3/1, Bit Slice2/1, Bit Slice1/1, Bit Slice/1
  concatenate/1 -> Out1/1

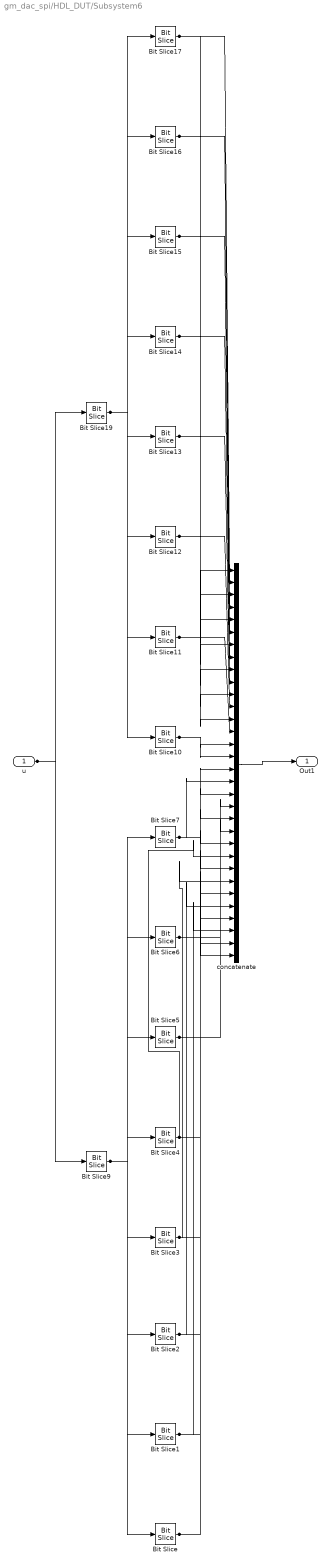
== system gm_dac_spi/HDL_DUT/Subsystem6 ==
  u : Inport  OutDataTypeStr=int16  PortDimensions=1  SampleTime=3.2e-07
  Bit Slice : hdlsllib/Logic and Bit Operations/Bit Slice  lidx=double(0)  ridx=double(0)
      settings: SourceProductBaseCode=SL
  Bit Slice1 : hdlsllib/Logic and Bit Operations/Bit Slice  lidx=double(1)  ridx=double(1)
      settings: SourceProductBaseCode=SL
  Bit Slice10 : hdlsllib/Logic and Bit Operations/Bit Slice  lidx=double(0)  ridx=double(0)
      settings: SourceProductBaseCode=SL
  Bit Slice11 : hdlsllib/Logic and Bit Operations/Bit Slice  lidx=double(1)  ridx=double(1)
      settings: SourceProductBaseCode=SL
  Bit Slice12 : hdlsllib/Logic and Bit Operations/Bit Slice  lidx=double(2)  ridx=double(2)
      settings: SourceProductBaseCode=SL
  Bit Slice13 : hdlsllib/Logic and Bit Operations/Bit Slice  lidx=double(3)  ridx=double(3)
      settings: SourceProductBaseCode=SL
  Bit Slice14 : hdlsllib/Logic and Bit Operations/Bit Slice  lidx=double(4)  ridx=double(4)
      settings: SourceProductBaseCode=SL
  Bit Slice15 : hdlsllib/Logic and Bit Operations/Bit Slice  lidx=double(5)  ridx=double(5)
      settings: SourceProductBaseCode=SL
  Bit Slice16 : hdlsllib/Logic and Bit Operations/Bit Slice  lidx=double(6)  ridx=double(6)
      settings: SourceProductBaseCode=SL
  Bit Slice17 : hdlsllib/Logic and Bit Operations/Bit Slice  lidx=double(7)  ridx=double(7)
      settings: SourceProductBaseCode=SL
  Bit Slice19 : hdlsllib/Logic and Bit Operations/Bit Slice  lidx=double(15)  ridx=double(8)
      settings: SourceProductBaseCode=SL
  Bit Slice2 : hdlsllib/Logic and Bit Operations/Bit Slice  lidx=double(2)  ridx=double(2)
      settings: SourceProductBaseCode=SL
  Bit Slice3 : hdlsllib/Logic and Bit Operations/Bit Slice  lidx=double(3)  ridx=double(3)
      settings: SourceProductBaseCode=SL
  Bit Slice4 : hdlsllib/Logic and Bit Operations/Bit Slice  lidx=double(4)  ridx=double(4)
      settings: SourceProductBaseCode=SL
  Bit Slice5 : hdlsllib/Logic and Bit Operations/Bit Slice  lidx=double(5)  ridx=double(5)
      settings: SourceProductBaseCode=SL
  Bit Slice6 : hdlsllib/Logic and Bit Operations/Bit Slice  lidx=double(6)  ridx=double(6)
      settings: SourceProductBaseCode=SL
  Bit Slice7 : hdlsllib/Logic and Bit Operations/Bit Slice  lidx=double(7)  ridx=double(7)
      settings: SourceProductBaseCode=SL
  Bit Slice9 : hdlsllib/Logic and Bit Operations/Bit Slice  lidx=double(7)  ridx=double(0)
      settings: SourceProductBaseCode=SL
  concatenate : Concatenate  NumInputs=32
  Out1 : Outport  SampleTime=3.2e-07
  wires:
  u/1 -> Bit Slice9/1, Bit Slice19/1
  Bit Slice/1 -> concatenate/32, concatenate/31
  Bit Slice1/1 -> concatenate/30, concatenate/29
  Bit Slice10/1 -> concatenate/16, concatenate/15
  Bit Slice11/1 -> concatenate/14, concatenate/13
  Bit Slice12/1 -> concatenate/12, concatenate/11
  Bit Slice13/1 -> concatenate/10, concatenate/9
  Bit Slice14/1 -> concatenate/8, concatenate/7
  Bit Slice15/1 -> concatenate/6, concatenate/5
  Bit Slice16/1 -> concatenate/4, concatenate/3
  Bit Slice17/1 -> concatenate/2, concatenate/1
  Bit Slice19/1 -> Bit Slice17/1, Bit Slice16/1, Bit Slice15/1, Bit Slice14/1, Bit Slice13/1, Bit Slice12/1, Bit Slice11/1, Bit Slice10/1
  Bit Slice2/1 -> concatenate/28, concatenate/27
  Bit Slice3/1 -> concatenate/26, concatenate/25
  Bit Slice4/1 -> concatenate/24, concatenate/23
  Bit Slice5/1 -> concatenate/22, concatenate/21
  Bit Slice6/1 -> concatenate/20, concatenate/19
  Bit Slice7/1 -> concatenate/18, concatenate/17
  Bit Slice9/1 -> Bit Slice7/1, Bit Slice6/1, Bit Slice5/1, Bit Slice4/1, Bit Slice3/1, Bit Slice2/1, Bit Slice1/1, Bit Slice/1
  concatenate/1 -> Out1/1

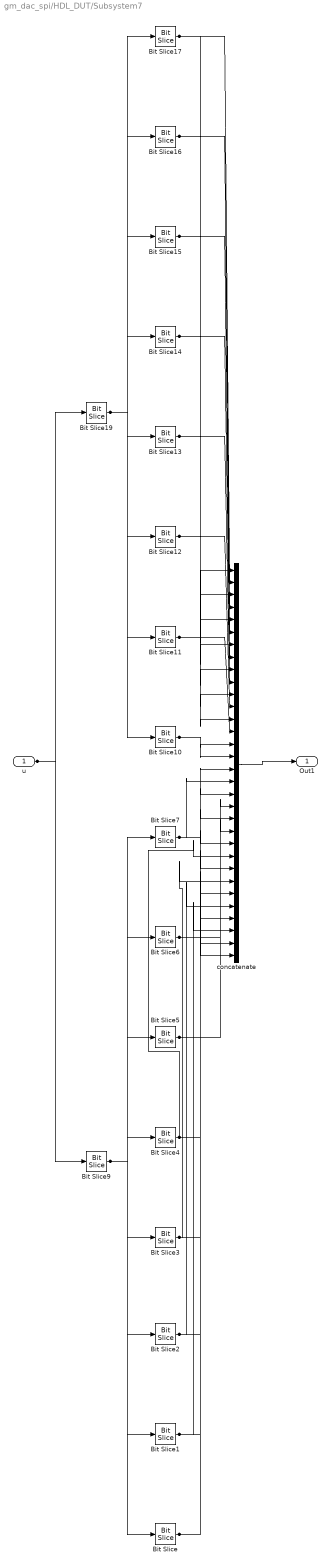
== system gm_dac_spi/HDL_DUT/Subsystem7 ==
  u : Inport  OutDataTypeStr=int16  PortDimensions=1  SampleTime=3.2e-07
  Bit Slice : hdlsllib/Logic and Bit Operations/Bit Slice  lidx=double(0)  ridx=double(0)
      settings: SourceProductBaseCode=SL
  Bit Slice1 : hdlsllib/Logic and Bit Operations/Bit Slice  lidx=double(1)  ridx=double(1)
      settings: SourceProductBaseCode=SL
  Bit Slice10 : hdlsllib/Logic and Bit Operations/Bit Slice  lidx=double(0)  ridx=double(0)
      settings: SourceProductBaseCode=SL
  Bit Slice11 : hdlsllib/Logic and Bit Operations/Bit Slice  lidx=double(1)  ridx=double(1)
      settings: SourceProductBaseCode=SL
  Bit Slice12 : hdlsllib/Logic and Bit Operations/Bit Slice  lidx=double(2)  ridx=double(2)
      settings: SourceProductBaseCode=SL
  Bit Slice13 : hdlsllib/Logic and Bit Operations/Bit Slice  lidx=double(3)  ridx=double(3)
      settings: SourceProductBaseCode=SL
  Bit Slice14 : hdlsllib/Logic and Bit Operations/Bit Slice  lidx=double(4)  ridx=double(4)
      settings: SourceProductBaseCode=SL
  Bit Slice15 : hdlsllib/Logic and Bit Operations/Bit Slice  lidx=double(5)  ridx=double(5)
      settings: SourceProductBaseCode=SL
  Bit Slice16 : hdlsllib/Logic and Bit Operations/Bit Slice  lidx=double(6)  ridx=double(6)
      settings: SourceProductBaseCode=SL
  Bit Slice17 : hdlsllib/Logic and Bit Operations/Bit Slice  lidx=double(7)  ridx=double(7)
      settings: SourceProductBaseCode=SL
  Bit Slice19 : hdlsllib/Logic and Bit Operations/Bit Slice  lidx=double(15)  ridx=double(8)
      settings: SourceProductBaseCode=SL
  Bit Slice2 : hdlsllib/Logic and Bit Operations/Bit Slice  lidx=double(2)  ridx=double(2)
      settings: SourceProductBaseCode=SL
  Bit Slice3 : hdlsllib/Logic and Bit Operations/Bit Slice  lidx=double(3)  ridx=double(3)
      settings: SourceProductBaseCode=SL
  Bit Slice4 : hdlsllib/Logic and Bit Operations/Bit Slice  lidx=double(4)  ridx=double(4)
      settings: SourceProductBaseCode=SL
  Bit Slice5 : hdlsllib/Logic and Bit Operations/Bit Slice  lidx=double(5)  ridx=double(5)
      settings: SourceProductBaseCode=SL
  Bit Slice6 : hdlsllib/Logic and Bit Operations/Bit Slice  lidx=double(6)  ridx=double(6)
      settings: SourceProductBaseCode=SL
  Bit Slice7 : hdlsllib/Logic and Bit Operations/Bit Slice  lidx=double(7)  ridx=double(7)
      settings: SourceProductBaseCode=SL
  Bit Slice9 : hdlsllib/Logic and Bit Operations/Bit Slice  lidx=double(7)  ridx=double(0)
      settings: SourceProductBaseCode=SL
  concatenate : Concatenate  NumInputs=32
  Out1 : Outport  SampleTime=3.2e-07
  wires:
  u/1 -> Bit Slice9/1, Bit Slice19/1
  Bit Slice/1 -> concatenate/32, concatenate/31
  Bit Slice1/1 -> concatenate/30, concatenate/29
  Bit Slice10/1 -> concatenate/16, concatenate/15
  Bit Slice11/1 -> concatenate/14, concatenate/13
  Bit Slice12/1 -> concatenate/12, concatenate/11
  Bit Slice13/1 -> concatenate/10, concatenate/9
  Bit Slice14/1 -> concatenate/8, concatenate/7
  Bit Slice15/1 -> concatenate/6, concatenate/5
  Bit Slice16/1 -> concatenate/4, concatenate/3
  Bit Slice17/1 -> concatenate/2, concatenate/1
  Bit Slice19/1 -> Bit Slice17/1, Bit Slice16/1, Bit Slice15/1, Bit Slice14/1, Bit Slice13/1, Bit Slice12/1, Bit Slice11/1, Bit Slice10/1
  Bit Slice2/1 -> concatenate/28, concatenate/27
  Bit Slice3/1 -> concatenate/26, concatenate/25
  Bit Slice4/1 -> concatenate/24, concatenate/23
  Bit Slice5/1 -> concatenate/22, concatenate/21
  Bit Slice6/1 -> concatenate/20, concatenate/19
  Bit Slice7/1 -> concatenate/18, concatenate/17
  Bit Slice9/1 -> Bit Slice7/1, Bit Slice6/1, Bit Slice5/1, Bit Slice4/1, Bit Slice3/1, Bit Slice2/1, Bit Slice1/1, Bit Slice/1
  concatenate/1 -> Out1/1
